simulink subsystem "MPC12_nlpsol"  (R2022b)
settings: Solver=VariableStepAuto  StartTime=0.0  StopTime=10.0  RelTol=1e-3
undefined symbols (not defined in the file): param_jointspace_ct, param_MPC12, param_robot, param_traj_data, param_weight_init
settings Model: Creator=emu  LastModifiedBy=emu
settings OptimizationCC: ReuseModelBlockBuffer=on

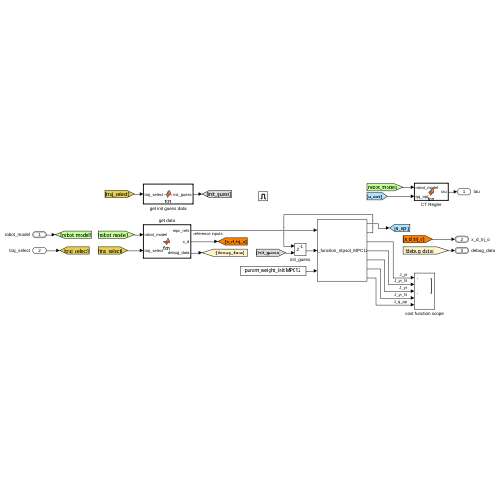
[thumbnail: Simulink's stored preview of the top-level diagram]
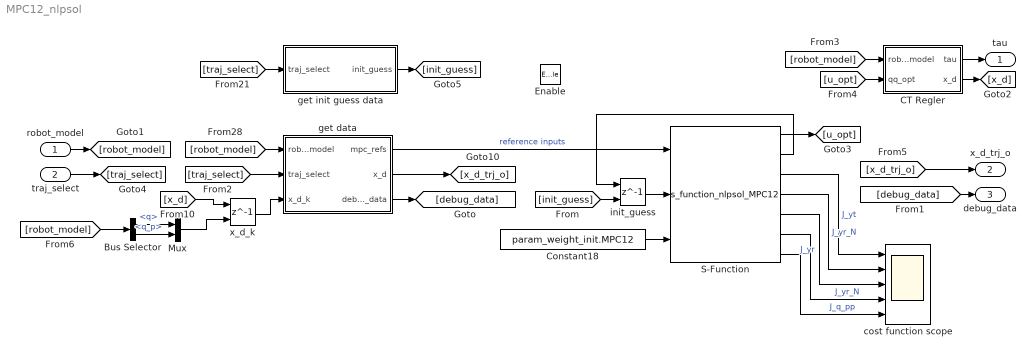
== system MPC12_nlpsol ==
  robot_model : Inport  OutDataTypeStr=Bus: robot_model
  traj_select : Inport  Port=2
  Enable : EnablePort
  Bus Selector : BusSelector  OutputSignals=q,q_p
  CT Regler : MATLAB Function  TreatAsAtomicUnit=on
  Constant18 : Constant  Value=param_weight_init.MPC12  VectorParams1D=off
  Mux : Mux  Inputs=2
  S-Function : S-Function  FunctionName=s_function_nlpsol_MPC12  Parameters='s_functions/ur5e_6dof/MPC12.casadi', 'MPC12'  SFunctionModules='MPC12'  SFunctionDeploymentMode=off  EnableBusSupport=off
  cost function scope : Scope  NumInputPorts=5
  get data : MATLAB Function  TreatAsAtomicUnit=on
  get init guess data : MATLAB Function  TreatAsAtomicUnit=on
  init_guess : Delay  DelayLength=1  InitialConditionSource=Input port  InitialCondition=1
      settings: InputPortMap=u0,p4
  x_d_k : Delay  DelayLength=1  InitialConditionSource=Input port  InitialCondition=1
      settings: InputPortMap=u0,p4
  tau : Outport
  x_d_trj_o : Outport  Port=2  OutDataTypeStr=Bus: x_d
  debug_data : Outport  Port=3  OutDataTypeStr=Bus: debug_data_bus
  wires:
  S-Function/2 -> init_guess/1
  S-Function/7 -> cost function scope/5  "J_q_pp"
  [debug_data] -> debug_data/1
  get data/1(mpc_refs) -> S-Function/1  "reference inputs"
  [robot_model] -> get data/1(robot_model)
  get data/2(x_d) -> [x_d_trj_o]
  [traj_select] -> get init guess data/1(traj_select)
  [init_guess] -> init_guess/2
  CT Regler/1(tau) -> tau/1
  S-Function/6 -> cost function scope/4  "J_yr_N"
  traj_select/1 -> [traj_select]
  [u_opt] -> CT Regler/2(qq_opt)
  S-Function/4 -> cost function scope/2  "J_yr_N"
  [traj_select] -> get data/2(traj_select)
  [robot_model] -> CT Regler/1(robot_model)
  robot_model/1 -> [robot_model]
  init_guess/1 -> S-Function/2
  get init guess data/1(init_guess) -> [init_guess]
  get data/3(debug_data) -> [debug_data]
  Constant18/1 -> S-Function/3
  S-Function/3 -> cost function scope/1  "J_yt"
  S-Function/5 -> cost function scope/3  "J_yr"
  [x_d_trj_o] -> x_d_trj_o/1
  S-Function/1 -> [u_opt]
  [robot_model] -> Bus Selector/1
  [x_d] -> x_d_k/1
  x_d_k/1 -> get data/3(x_d_k)
  CT Regler/2(x_d) -> [x_d]
  Bus Selector/1 -> Mux/1  "<q>"
  Bus Selector/2 -> Mux/2  "<q_p>"
  Mux/1 -> x_d_k/2

== matlab function MPC12_nlpsol/CT Regler ==
  data: robot_model input Bus: robot_model; tau output; qq_opt input; param_robot parameter; param_jointspace_ct parameter; x_d output
function [tau, x_d] = fcn(robot_model, qq_opt, param_robot, param_jointspace_ct)

n = param_robot.n_DOF;
q = robot_model.q_noise;      % generalized coordinates
q_p = robot_model.q_p_noise;  % time derivative of generalized coordinates

if size(qq_opt, 2) ~= 0 && size(qq_opt, 1) ~= 1
    
    q_d_0 = qq_opt(1:n, 1); % q_0
    q_d_0_p = qq_opt(n+1:2*n, 1); %q_p_0
    q_d_0_pp = qq_opt(2*n+1:3*n, 1); %q_p_00
    
    M = robot_model.M;      % inertia matrix
    C_rnea = robot_model.C_rnea; % C_rnea(q, q_p) = C(q, q_p)q_p + g(q) = n(q, q_p)
    
    e = q - q_d_0;
    e_p = q_p - q_d_0_p;
    
    K_D_q = param_jointspace_ct.MPC12.K_D_q;
    K_P_q = param_jointspace_ct.MPC12.K_P_q;
    tau = M*(q_d_0_pp - K_D_q * e_p - K_P_q * e) + C_rnea;

    q_d_1 = qq_opt(1+3*n:4*n, 1); % q_0
    q_d_1_p = qq_opt(1+4*n:5*n, 1); %q_p_0

    x_d = [q_d_1; q_d_1_p];
else
    tau = zeros(n,1);
    x_d = [q; q_p];
end

== matlab function MPC12_nlpsol/get data ==
  settings: updateMethod=DISCRETE  sampleTime=param_global.Ta
  data: mpc_refs output; robot_model input Bus: robot_model; param_MPC12 parameter; x_d output Bus: x_d; debug_data output Bus: debug_data_bus; param_traj_data parameter; traj_select input; x_d_k input
function [mpc_refs, x_d, debug_data] = fcn(robot_model, param_MPC12, param_traj_data, traj_select, x_d_k)
persistent cnt;

if(isempty(cnt))
    cnt = 1;
end

param_MPC = param_MPC12;
N         = param_MPC.N;
N_step    = param_MPC.N_step;

% Parameters
q    = robot_model.q;      % generalized coordinates
q_p  = robot_model.q_p;  % time derivative of generalized coordinates
q_pp = robot_model.q_pp;
H    = robot_model.H;
J    = robot_model.J;
J_p  = robot_model.J_p;

R = H(1:3,1:3);% desired Orientation as rotational matrix
R_d = param_traj_data.R_d(:,:, cnt, traj_select);
q_d = param_traj_data.q_d(:, cnt, traj_select);

%y_q_err = quat_mult(y_q_e, quat_inv(param_traj_data.q_d(1:4, cnt, traj_select)));
q_err = rotm2quat_v4(R*R_d');
%y_q_e = rotm2quat_v4(R);
q_e = quat_mult(q_d, q_err);

% Current Pose of Endeffector
y = [H(1:3,4); q_e];
y_p = J*q_p;
y_pp = J*q_pp + J_p*q_p;

%x_k = [q;q_p]; das ist hier nicht der Fall, open loop!
x_k = x_d_k; % open loop mpc

% Assemble vector of recieved output measurements
p_d     = param_traj_data.p_d(   1:3, cnt : N_step : cnt + (N)*N_step, traj_select);
q_d     = param_traj_data.q_d(   1:4, cnt : N_step : cnt + (N)*N_step, traj_select);

omega_d   = param_traj_data.omega_d(  1:3, cnt : N_step : cnt + (N-1)*N_step, traj_select);
omega_d_p = param_traj_data.omega_d_p(1:3, cnt : N_step : cnt + (N-1)*N_step, traj_select);

alpha_d    = param_traj_data.alpha_d(           :, cnt : N_step : cnt + (N)*N_step, traj_select);
alpha_d_p  = param_traj_data.alpha_d_p(         :, cnt : N_step : cnt + (N)*N_step, traj_select);
alpha_d_pp = param_traj_data.alpha_d_pp(        :, cnt : N_step : cnt + (N)*N_step, traj_select);
rot_ax_d   = param_traj_data.rot_ax_d(          :, cnt : N_step : cnt + (N)*N_step, traj_select);
alpha_d_offset = param_traj_data.alpha_d_offset(:, cnt : N_step : cnt + (N)*N_step, traj_select);
q_d_rel = param_traj_data.q_d_rel(              :, cnt : N_step : cnt + (N)*N_step, traj_select);

if(N_step == 1)
    y_d = [p_d; q_d];
else
    p_d_kp1 = param_traj_data.p_d(   1:3, cnt+1:cnt+2, traj_select);
    q_d_kp1 = param_traj_data.q_d(   1:4, cnt+1:cnt+2, traj_select);
    y_d     = [[p_d(:,1), p_d_kp1, p_d(:,2:end-2)]; [q_d(:,1), q_d_kp1, q_d(:,2:end-2)]];
end

%% Reference out
mpc_refs = [x_k(:); y_d(:)];

%% TRAJECTORY OUT
x_d.p_d       = param_traj_data.p_d(1:3, cnt , traj_select);    %y0
x_d.p_d_p     = param_traj_data.p_d_p(1:3, cnt , traj_select);  %y0p
x_d.p_d_pp    = param_traj_data.p_d_pp(1:3, cnt , traj_select); %y0pp
x_d.Phi_d     = param_traj_data.Phi_d(:, cnt , traj_select);
x_d.Phi_d_p   = param_traj_data.Phi_d_p(:, cnt, traj_select);
x_d.Phi_d_pp  = param_traj_data.Phi_d_pp(:,cnt, traj_select);
x_d.R_d       = R_d;
x_d.q_d       = q_d(1:4, 1);
x_d.q_d_p     = param_traj_data.q_d_p(1:4, cnt, traj_select);
x_d.q_d_pp    = param_traj_data.q_d_pp(1:4, cnt, traj_select);
x_d.omega_d   = omega_d(1:3, 1);
x_d.omega_d_p = omega_d_p(1:3, 1);
x_d.alpha_d    = alpha_d(:, 1);
x_d.alpha_d_p  = alpha_d_p(:, 1);
x_d.alpha_d_pp = alpha_d_pp(:, 1);
x_d.rot_ax_d   = rot_ax_d(:, 1);
x_d.alpha_d_offset = alpha_d_offset(:, 1);
x_d.q_d_rel = q_d_rel(:, 1);

%% DEBUG
debug_data.p           = y(1:3);
debug_data.p_p         = y_p(1:3);
debug_data.p_pp        = y_pp(1:3);
debug_data.Phi     = rotm2eul_v2(R);
debug_data.Phi_p   = [0; 0; 0]; % ?????? Phi_p = T * omega?
debug_data.Phi_pp  = [0; 0; 0]; % ??????
debug_data.q           = y(4:7);
debug_data.omega       = y_p(4:6);
debug_data.omega_p     = y_pp(4:6);
debug_data.p_err       = y(1:3) - param_traj_data.p_d(:, cnt, traj_select);
debug_data.p_p_err     = y_p(1:3) - param_traj_data.p_d_p(:, cnt, traj_select);
debug_data.p_pp_err    = y_pp(1:3) - param_traj_data.p_d_pp(:, cnt, traj_select);
debug_data.q_err       = q_err;
debug_data.omega_err   = y_p(4:6)  - omega_d(1:3, 1);
debug_data.omega_p_err = y_pp(4:6) - omega_d_p(1:3, 1);

cnt = cnt+1;

== matlab function MPC12_nlpsol/get init guess data ==
  data: traj_select input; param_MPC12_init_guess parameter; init_guess output
function init_guess   = fcn(traj_select, param_MPC12_init_guess)

%init_guess = param_MPC12_init_guess.init_guess(1,:);
init_guess = param_MPC12_init_guess.init_guess(traj_select,:);
